simulink model "MonoRail_APU_Complete_R2016"  (R2016a)
settings: Solver=ode1  StartTime=0.0  StopTime=4.00  FixedStep=1e-6  MaxStep=1e-4  RelTol=1e-3
libraries: powerlib x67, powerlib_meascontrol x19, simulink x9, simulink_extras x3
settings Model: Creator=Hirect_MKTG  LastModifiedBy=Testinglaptop2
settings SimscapeCC: SimscapeNormalizeSystem=off

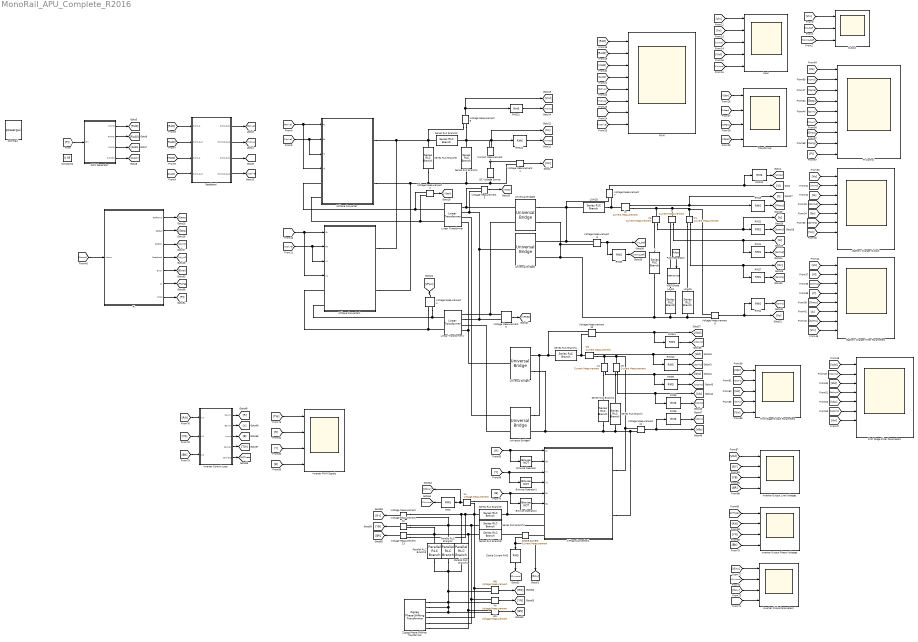
== system MonoRail_APU_Complete_R2016 ==
  3 Phase Converter : Subsystem
  3 Phase Converter1 : Subsystem
  3 Phase Converter2 : Subsystem
  BN : powerlib/Measurements/Voltage Measurement  PhasorSimulation=off  OutputType=Complex  PSBequivalent=0
  Battery Charger Filter Parameters : Scope  NumInputPorts=8
  Battery Charger Output : Scope  NumInputPorts=8
  Bitwise Operator : simulink/Logic and Bit Operations/Bitwise Operator  logicop=NOT  UseBitMask=off  BitMask=bin2dec('11011001')  BitMaskRealWorld=Stored Integer
  Bitwise Operator1 : simulink/Logic and Bit Operations/Bitwise Operator  logicop=NOT  UseBitMask=off  BitMask=bin2dec('11011001')  BitMaskRealWorld=Stored Integer
  Bitwise Operator2 : simulink/Logic and Bit Operations/Bitwise Operator  logicop=NOT  UseBitMask=off  BitMask=bin2dec('11011001')  BitMaskRealWorld=Stored Integer
  C : powerlib/Elements/Series RLC Branch  LConnTagsString=__new0  RConnTagsString=__new0  BranchType=C  Resistance=1  Inductance=1e-3  SetiL0=off  InitialCurrent=0  Capacitance=20e-3  Setx0=off  InitialVoltage=0  Measurements=None
  Choke Current RMS : powerlib_meascontrol/Measurements/RMS  TrueRMS=on  Freq=60  RMSInit=120  Ts=0
  Choke Current : powerlib/Measurements/Current Measurement  PhasorSimulation=off  OutputType=Complex  PSBequivalent=0
  Constant2 : Constant  Value=0.95  VectorParams1D=off
  Current Measurement5 : powerlib/Measurements/Current Measurement  PhasorSimulation=off  OutputType=Complex  PSBequivalent=0
  DC Voltage Source : powerlib/Electrical Sources/DC Voltage Source  Amplitude=500  Measurements=None
  Deadband : Subsystem
  First Stage Filter Parameters : Scope  NumInputPorts=8
  "First Stage Output Parameters " : Scope  NumInputPorts=5
  IGBT/Diode : powerlib/Power Electronics/IGBT//Diode  Ron=1e-3  Rs=1e5  Cs=inf  Measurements=on
  Input : Scope  NumInputPorts=5
  Inverter Choke Parameters : Scope  NumInputPorts=4
  Inverter Control Loop : Subsystem
  Inverter Output Line Voltages : Scope  NumInputPorts=4
  Inverter Output Phase Voltages : Scope  NumInputPorts=4
  Inverter PWM Signals : Scope  NumInputPorts=4
  Io : powerlib/Measurements/Current Measurement  PhasorSimulation=off  OutputType=Complex  PSBequivalent=0
  Ir{,1..5} (6 alike) : powerlib/Measurements/Current Measurement  PhasorSimulation=off  OutputType=Complex  PSBequivalent=0
  LOAD : powerlib/Elements/Series RLC Branch  LConnTagsString=__new0  RConnTagsString=__new0  BranchType=R  Resistance=58e-03  Inductance=1e-3  SetiL0=off  InitialCurrent=0  Capacitance=1e-6  Setx0=off  InitialVoltage=0  Measurements=None
  LOAD1 : powerlib/Elements/Series RLC Branch  LConnTagsString=__new0  RConnTagsString=__new0  BranchType=R  Resistance=1  Inductance=1e-3  SetiL0=off  InitialCurrent=0  Capacitance=1e-6  Setx0=off  InitialVoltage=0  Measurements=None
  LOAD3 : powerlib/Elements/Series RLC Branch  LConnTagsString=__new0  RConnTagsString=__new0  BranchType=L  Resistance=77e-03  Inductance=100e-6  SetiL0=off  InitialCurrent=0  Capacitance=1e-6  Setx0=off  InitialVoltage=0  Measurements=None
  Linear Transformer : powerlib/Elements/Linear Transformer  UNITS=SI  NominalPower=[ 50e3 50 ]  winding1=[1000 0 0]  winding2=[28.42 0 0]  ThreeWindings=on  winding3=[781 0 0]  RmLm=[inf inf]  Measurements=None  DataType=on
  Linear Transformer1 : powerlib/Elements/Linear Transformer  UNITS=SI  NominalPower=[ 50e3 50 ]  winding1=[1000 0 0]  winding2=[28.42 0 0]  ThreeWindings=on  winding3=[781 0 0]  RmLm=[inf inf]  Measurements=None  DataType=on
  Output : Scope  NumInputPorts=3
  PI : Subsystem
  PI Control : Scope  NumInputPorts=9
  PWM : Scope  NumInputPorts=8
  PWM Generator : Subsystem
  Parallel RLC Branch1 : powerlib/Elements/Parallel RLC Branch  LConnTagsString=a  RConnTagsString=__new0  BranchType=RC  Resistance=7.5  Inductance=1e-3  SetiL0=off  InitialCurrent=0  Capacitance=30e-06  Setx0=off  InitialVoltage=0  Measurements=None
  Parallel RLC Branch2 : powerlib/Elements/Parallel RLC Branch  LConnTagsString=a  RConnTagsString=__new0  BranchType=RC  Resistance=7.5  Inductance=1e-3  SetiL0=off  InitialCurrent=0  Capacitance=30e-06  Setx0=off  InitialVoltage=0  Measurements=None
  Parallel RLC Branch3 : powerlib/Elements/Parallel RLC Branch  LConnTagsString=a  RConnTagsString=__new0  BranchType=RC  Resistance=7.5  Inductance=1e-3  SetiL0=off  InitialCurrent=0  Capacitance=30e-06  Setx0=off  InitialVoltage=0  Measurements=None
  Pulse Generator : DiscretePulseGenerator  Period=1e06  PulseWidth=1e06  SampleTime=1e-06
  RMS{,1..14} (15 alike) : powerlib_meascontrol/Measurements/RMS  TrueRMS=on  Freq=60  RMSInit=120  Ts=0
  RN : powerlib/Measurements/Voltage Measurement  PhasorSimulation=off  OutputType=Complex  PSBequivalent=0
  Series RLC Branch : powerlib/Elements/Series RLC Branch  LConnTagsString=__new0  RConnTagsString=__new0  BranchType=R  Resistance=12.25  Inductance=1e-3  SetiL0=off  InitialCurrent=0  Capacitance=1e-6  Setx0=off  InitialVoltage=0  Measurements=None
  Series RLC Branch1 : powerlib/Elements/Series RLC Branch  LConnTagsString=__new0  RConnTagsString=__new0  BranchType=L  Resistance=12.25  Inductance=1e-3  SetiL0=off  InitialCurrent=0  Capacitance=1e-6  Setx0=off  InitialVoltage=0  Measurements=None
  Series RLC Branch2 : powerlib/Elements/Series RLC Branch  LConnTagsString=__new0  RConnTagsString=__new0  BranchType=C  Resistance=12.25  Inductance=1e-3  SetiL0=off  InitialCurrent=0  Capacitance=225e-6  Setx0=off  InitialVoltage=0  Measurements=None
  Series RLC Branch3 : powerlib/Elements/Series RLC Branch  LConnTagsString=__new0  RConnTagsString=__new0  BranchType=L  Resistance=12.25  Inductance=0.5e-3  SetiL0=off  InitialCurrent=0  Capacitance=1e-6  Setx0=off  InitialVoltage=0  Measurements=None
  Series RLC Branch4 : powerlib/Elements/Series RLC Branch  LConnTagsString=__new0  RConnTagsString=__new0  BranchType=RC  Resistance=0.1  Inductance=1e-3  SetiL0=off  InitialCurrent=0  Capacitance=225e-6  Setx0=off  InitialVoltage=0  Measurements=None
  Series RLC Branch5 : powerlib/Elements/Series RLC Branch  LConnTagsString=__new0  RConnTagsString=__new0  BranchType=C  Resistance=12.25  Inductance=1e-3  SetiL0=off  InitialCurrent=0  Capacitance=225e-6  Setx0=off  InitialVoltage=0  Measurements=None
  Series RLC Branch6 : powerlib/Elements/Series RLC Branch  LConnTagsString=__new0  RConnTagsString=__new0  BranchType=L  Resistance=1  Inductance=0.85e-3  SetiL0=off  InitialCurrent=0  Capacitance=1e-6  Setx0=off  InitialVoltage=0  Measurements=None
  Series RLC Branch7 : powerlib/Elements/Series RLC Branch  LConnTagsString=__new0  RConnTagsString=__new0  BranchType=L  Resistance=1  Inductance=0.85e-3  SetiL0=off  InitialCurrent=0  Capacitance=1e-6  Setx0=off  InitialVoltage=0  Measurements=None
  Series RLC Branch8 : powerlib/Elements/Series RLC Branch  LConnTagsString=__new0  RConnTagsString=__new0  BranchType=L  Resistance=1  Inductance=0.85e-3  SetiL0=off  InitialCurrent=0  Capacitance=1e-6  Setx0=off  InitialVoltage=0  Measurements=None
  Transformer : Scope  NumInputPorts=4
  Universal Bridge1 : powerlib/Power Electronics/Universal Bridge  Arms=1  SnubberResistance=1e5  SnubberCapacitance=inf  Device=Diodes  Ron=1e-3  Lon=0  ForwardVoltages="[  0  0  ]"  ForwardVoltage=0  GTOparameters=[ 10e-6 , 20e-6 ]  IGBTparameters=[ 1e-6 , 2e-6 ]  Measurements=None  Measurements_2=None  converterType=Rectifier
  Universal Bridge2 : powerlib/Power Electronics/Universal Bridge  Arms=1  SnubberResistance=1e5  SnubberCapacitance=inf  Device=Diodes  Ron=1e-3  Lon=0  ForwardVoltages="[  0  0  ]"  ForwardVoltage=0  GTOparameters=[ 10e-6 , 20e-6 ]  IGBTparameters=[ 1e-6 , 2e-6 ]  Measurements=None  Measurements_2=None  converterType=Rectifier
  Universal Bridge3 : powerlib/Power Electronics/Universal Bridge  Arms=2  SnubberResistance=1e5  SnubberCapacitance=inf  Device=Diodes  Ron=1e-3  Lon=0  ForwardVoltages="[  0  0  ]"  ForwardVoltage=0  GTOparameters=[ 10e-6 , 20e-6 ]  IGBTparameters=[ 1e-6 , 2e-6 ]  Measurements=None  Measurements_2=None  converterType=Rectifier
  Universal Bridge4 : powerlib/Power Electronics/Universal Bridge  Arms=2  SnubberResistance=1e5  SnubberCapacitance=inf  Device=Diodes  Ron=1e-3  Lon=0  ForwardVoltages="[  0  0  ]"  ForwardVoltage=0  GTOparameters=[ 10e-6 , 20e-6 ]  IGBTparameters=[ 1e-6 , 2e-6 ]  Measurements=None  Measurements_2=None  converterType=Rectifier
  VL : powerlib/Measurements/Voltage Measurement  PhasorSimulation=off  OutputType=Complex  PSBequivalent=0
  Voltage Measurement{,1..13} (14 alike) : powerlib/Measurements/Voltage Measurement  PhasorSimulation=off  OutputType=Complex  PSBequivalent=0
  YN : powerlib/Measurements/Voltage Measurement  PhasorSimulation=off  OutputType=Complex  PSBequivalent=0
  Zigzag Phase-Shifting Transformer : powerlib/Elements/Zigzag Phase-Shifting Transformer  SecondaryConnection=Yg  SetSaturation=off  SetInitialFlux=off  Measurements=None  UNITS=pu  NominalPower=[ 100e6 60]  PrimaryVoltage=10e3  SecondaryVoltage="[ 30e3  +15]"  Winding1=[ 0.002 0.08 ]  Winding2="[ 0.002  0.08 ]"  Winding3=[ 0.002 0.08 ]  RmLm=[ 500 500 ]  Rm=500  Saturation=[ 0,0 ; 0.0024,1.2 ; 1.0,1.52 ]  InitialFluxes=[0,0,0]  BreakLoop=off  DiscreteSolver=Trapezoidal iterative  DataType=off
  powergui : powerlib/powergui  Priority=1  SimulationMode=Discrete  SampleTime=1e-6  frequency=60  Iterations=50  frequencyindice=0  Pbase=100e6  ErrMax=1e-4  UnitsV=kV  UnitsW=MW  buscounter=0  FunctionMessages=off  echomessages=off  EnableUseOfTLC=off  CurrentSourceSwitches=off  DisableSnubberDevices=off  DisableRonSwitches=off  DisableVfSwitches=off  DisplayEquations=off  AutomaticDiscreteSolvers=off  SolverType=Tustin/Backward Euler (TBE)  Interpol=off  ExternalGateDelay=off  methode=off  Ts=100  x0status=blocks  SPID=on  SwTol=0  HookPort=off  NonlinearTolerance=1e-4  nMaxIteration=100  ContinueOnMaxIteration=off  RestoreLinks=warning  ResistiveCurrentMeasurement=off  Frange=[0:2:500]  Ylog=off  Xlog=on  ShowGrid=off  save=off  variable=ZData  structure=ScopeData1  ZoomFFT=on  StartTime=1  cycles=5  DisplayStyle=1  fundamental=50  FreqAxis=off  MaxFrequency=1000  frequencyindicesteady=1  RmsSteady=1  display=off
  wires:
  Current Measurement5/1 -> [Iin], RMS11/1
  Voltage Measurement1/1 -> [Vin]
  Voltage Measurement9/1 -> [Vinl], RMS12/1
  [Vo] -> PI Control/1
  [Vorms] -> PI Control/2
  [Step] -> PI Control/4
  Voltage Measurement7/1 -> [Vl], RMS10/1
  RMS10/1 -> [Vlrms]
  [Vin] -> Output/1
  [Vo_bef] -> Output/2
  [Vorms_bef] -> Output/3
  [Rdrive] -> 3 Phase Converter/4(Yb), 3 Phase Converter/1(Rt)
  [Ydrive] -> 3 Phase Converter/3(Yt), 3 Phase Converter/2(Rb)
  [Rpdrive] -> 3 Phase Converter1/1(Rt), 3 Phase Converter1/4(Yb)
  [Ypdrive] -> 3 Phase Converter1/2(Rb), 3 Phase Converter1/3(Yt)
  [Rd0] -> Deadband/1(PWM_0)
  [Rcd0] -> Deadband/2(PWM_0_C)
  [Rpd0] -> Deadband/3(PWM_P)
  [Rpcd0] -> Deadband/4(PWM_P_C)
  Deadband/1(PWM_0_D) -> [Rdrive]
  Deadband/2(PWM_0_C_D) -> [Ydrive]
  Deadband/3(PWM_P_D) -> [Rpdrive]
  Deadband/4(PWM_P_C_D) -> [Ypdrive]
  [Vin] -> Input/1
  RMS11/1 -> [Iinrms]
  [Iin] -> Input/2
  [Iinrms] -> Input/3
  RMS12/1 -> [Vinlrms]
  [Vinlrms] -> Input/5
  [Vinl] -> Input/4
  [Ramp] -> PI Control/3
  PWM Generator/1("PWM0 ") -> [Rd0]
  PWM Generator/2(PWMC) -> [Rcd0]
  PWM Generator/3(PWMP) -> [Rpd0]
  PWM Generator/4(PWMPC) -> [Rpcd0]
  PI/1(RefRamp) -> [Ramp]
  PI/2(RefSat) -> [Step]
  PI/3(RefCon) -> [ConIN]
  [Vorms] -> PI/1(Vorms)
  PI/5(Error) -> [Error]
  PI/6(PI) -> [PIorig]
  PI/7(PIsat) -> [PI]
  PI/4(Feedback) -> [Vo_un]
  [Rd0] -> PWM/1
  [Rcd0] -> PWM/2
  [Rpd0] -> PWM/3
  [Rpcd0] -> PWM/4
  [Rdrive] -> PWM/5
  [Ydrive] -> PWM/6
  [Rpdrive] -> PWM/7
  [Ypdrive] -> PWM/8
  Voltage Measurement2/1 -> [V0pri]
  Voltage Measurement3/1 -> [V0sec]
  Voltage Measurement5/1 -> [VPsec]
  Voltage Measurement4/1 -> [VPpri]
  [V0pri] -> Transformer/1
  [V0sec] -> Transformer/2
  [VPpri] -> Transformer/3
  [VPsec] -> Transformer/4
  [PI] -> PWM Generator/1(Phi)
  RMS7/1 -> [Ibrrms]
  Ir1/1 -> [Ibr], RMS7/1
  Pulse Generator/1 -> IGBT/Diode/1
  Ir/1 -> [Io], RMS1/1
  RMS1/1 -> [Iorms]
  RMS2/1 -> [Icrms]
  Ir2/1 -> [Ic], RMS2/1
  RMS3/1 -> [Ilrms]
  Io/1 -> RMS3/1, [Il]
  RMS4/1 -> [Vorms]
  Voltage Measurement6/1 -> [Vo], RMS4/1
  [Vo] -> Battery Charger Output/1
  [Vorms] -> Battery Charger Output/2
  [Io] -> Battery Charger Output/3
  [Iorms] -> Battery Charger Output/4
  [Ibr] -> Battery Charger Output/5
  [Ibrrms] -> Battery Charger Output/6
  Voltage Measurement8/1 -> [Vo_bef], RMS5/1
  RMS5/1 -> [Vorms_bef]
  [Vin] -> Battery Charger Output/7
  [Vo] -> Battery Charger Filter Parameters/1
  [Vlrms] -> Battery Charger Filter Parameters/3
  [Vl] -> Battery Charger Filter Parameters/2
  [Il] -> Battery Charger Filter Parameters/4
  [Ilrms] -> Battery Charger Filter Parameters/5
  [Ic] -> Battery Charger Filter Parameters/6
  [Icrms] -> Battery Charger Filter Parameters/7
  [Vo_un] -> PI Control/6
  [Error] -> PI Control/7
  [PIorig] -> PI Control/8
  [PI] -> PI Control/9
  [ConIN] -> PI Control/5
  Voltage Measurement10/1 -> RMS14/1, [Vdcl]
  RMS14/1 -> [Vdclrms]
  Ir3/1 -> RMS13/1, [Idcl]
  RMS13/1 -> [Idclrms]
  Ir4/1 -> RMS9/1, [Idcc]
  RMS9/1 -> [Idccrms]
  Ir5/1 -> RMS8/1, [Idc]
  RMS8/1 -> [Idcrms]
  Voltage Measurement11/1 -> RMS6/1, [Vdc]
  RMS6/1 -> [Vdcrms]
  [Vin] -> Battery Charger Filter Parameters/8
  [Vdcl] -> First Stage Filter Parameters/1
  [Vdclrms] -> First Stage Filter Parameters/2
  [Idcl] -> First Stage Filter Parameters/3
  [Idclrms] -> First Stage Filter Parameters/4
  [Idcc] -> First Stage Filter Parameters/5
  [Idccrms] -> First Stage Filter Parameters/6
  [Vin] -> First Stage Filter Parameters/7
  [Vin] -> "First Stage Output Parameters "/5
  [Vdc] -> "First Stage Output Parameters "/1
  [Vdcrms] -> "First Stage Output Parameters "/2
  [Idc] -> "First Stage Output Parameters "/3
  [Idcrms] -> "First Stage Output Parameters "/4
  Inverter Control Loop/5(Carrier2) -> [OPTheta]
  [Vlinv] -> Inverter Choke Parameters/1
  [B] -> Inverter PWM Signals/4
  [Y] -> Bitwise Operator1/1, 3 Phase Converter2/3(Yt)
  Bitwise Operator2/1 -> 3 Phase Converter2/6(Bb)
  [BN] -> Inverter Control Loop/3(In3)
  Inverter Control Loop/3(Ypwm) -> [B]
  Choke Current/1 -> Choke Current RMS/1, [Ilinv]
  [Y] -> Inverter PWM Signals/3
  [R] -> Bitwise Operator/1, 3 Phase Converter2/1(Rt)
  [TW] -> Inverter PWM Signals/1
  BN/1 -> [BN]
  [R] -> Inverter PWM Signals/2
  Inverter Control Loop/4(Carrier) -> [TW]
  [RN] -> Inverter Control Loop/1(In1)
  Inverter Control Loop/2(Bpwm) -> [Y]
  VL/1 -> [Vlinv], RMS/1
  [Ilinvrms] -> Inverter Choke Parameters/4
  RN/1 -> [RN]
  [OPTheta] -> Inverter Output Phase Voltages/1
  Voltage Measurement12/1 -> [YB]
  Bitwise Operator/1 -> 3 Phase Converter2/2(Rb)
  YN/1 -> [YN]
  [YN] -> Inverter Control Loop/2(In2)
  [BR] -> Inverter Output Line Voltages/4
  [Ilinv] -> Inverter Choke Parameters/3
  Voltage Measurement/1 -> [RY]
  [Vlinvrms] -> Inverter Choke Parameters/2
  [YB] -> Inverter Output Line Voltages/3
  Choke Current RMS/1 -> [Ilinvrms]
  Voltage Measurement13/1 -> [BR]
  [B] -> Bitwise Operator2/1, 3 Phase Converter2/5(Bt)
  Bitwise Operator1/1 -> 3 Phase Converter2/4(Yb)
  [RN] -> Inverter Output Phase Voltages/2
  [YN] -> Inverter Output Phase Voltages/3
  Inverter Control Loop/1(Rpwm) -> [R]
  [RY] -> Inverter Output Line Voltages/2
  [BN] -> Inverter Output Phase Voltages/4
  RMS/1 -> [Vlinvrms]
  [Vdcl] -> Inverter Output Line Voltages/1
  connections:
  3 Phase Converter1/RConn1 -- Series RLC Branch3/RConn1 -- Series RLC Branch5/LConn1 -- Voltage Measurement9/LConn2 -- 3 Phase Converter/RConn1
  3 Phase Converter1/RConn2 -- 3 Phase Converter/RConn2 -- Series RLC Branch5/RConn1 -- DC Voltage Source/LConn1 -- Voltage Measurement1/LConn2 -- Series RLC Branch4/RConn1
  Linear Transformer/LConn2 -- Voltage Measurement2/LConn2 -- 3 Phase Converter/LConn2
  3 Phase Converter1/LConn1 -- Linear Transformer1/LConn2 -- Voltage Measurement4/LConn2
  3 Phase Converter1/LConn2 -- Voltage Measurement4/LConn1 -- Linear Transformer1/LConn1
  3 Phase Converter/LConn1 -- Voltage Measurement2/LConn1 -- Linear Transformer/LConn1
  Series RLC Branch4/LConn1 -- Current Measurement5/RConn1 -- Series RLC Branch3/LConn1 -- Voltage Measurement9/LConn1
  DC Voltage Source/RConn1 -- Voltage Measurement1/LConn1 -- Current Measurement5/LConn1
  Universal Bridge3/LConn1 -- Linear Transformer/RConn1 -- Voltage Measurement3/LConn1
  Universal Bridge2/LConn1 -- Linear Transformer1/RConn2 -- Voltage Measurement5/LConn2 -- Voltage Measurement3/LConn2 -- Linear Transformer/RConn2
  Universal Bridge3/LConn2 -- Voltage Measurement5/LConn1 -- Linear Transformer1/RConn1
  LOAD3/RConn1 -- Universal Bridge3/RConn1 -- Voltage Measurement8/LConn1 -- Universal Bridge2/RConn1 -- Voltage Measurement7/LConn1
  Universal Bridge3/RConn2 -- C/RConn1 -- Voltage Measurement6/LConn2 -- LOAD1/RConn1 -- LOAD/RConn1 -- Universal Bridge2/RConn2 -- Voltage Measurement8/LConn2
  LOAD3/LConn1 -- Io/LConn1 -- Voltage Measurement7/LConn2
  Ir1/LConn1 -- Voltage Measurement6/LConn1 -- Ir/LConn1 -- Ir2/LConn1 -- Io/RConn1
  Ir1/RConn1 -- LOAD1/LConn1
  IGBT/Diode/RConn1 -- LOAD/LConn1
  IGBT/Diode/LConn1 -- Ir/RConn1
  Ir2/RConn1 -- C/LConn1
  Ir3/LConn1 -- Voltage Measurement10/LConn2 -- Series RLC Branch1/LConn1
  Universal Bridge4/RConn2 -- Universal Bridge1/RConn2 -- 3 Phase Converter2/RConn2 -- Voltage Measurement11/LConn2 -- Series RLC Branch/RConn1 -- Series RLC Branch2/RConn1
  Universal Bridge4/RConn1 -- Voltage Measurement10/LConn1 -- Series RLC Branch1/RConn1 -- Universal Bridge1/RConn1
  Universal Bridge1/LConn1 -- Linear Transformer/RConn4 -- Linear Transformer1/RConn4
  Universal Bridge4/LConn2 -- Linear Transformer1/RConn3
  Universal Bridge4/LConn1 -- Linear Transformer/RConn3
  Ir3/RConn1 -- 3 Phase Converter2/RConn1 -- Voltage Measurement11/LConn1 -- Ir5/LConn1 -- Ir4/LConn1
  Ir4/RConn1 -- Series RLC Branch2/LConn1
  Ir5/RConn1 -- Series RLC Branch/LConn1
  Zigzag Phase-Shifting Transformer/LConn2 -- BN/LConn2 -- Zigzag Phase-Shifting Transformer/LConn3 -- Parallel RLC Branch3/RConn1 -- Parallel RLC Branch1/RConn1 -- Parallel RLC Branch2/RConn1 -- RN/LConn2 -- YN/LConn2 -- Zigzag Phase-Shifting Transformer/LConn1
  Zigzag Phase-Shifting Transformer/LConn5 -- YN/LConn1 -- Series RLC Branch7/LConn1 -- Voltage Measurement/LConn2 -- Voltage Measurement12/LConn1 -- Parallel RLC Branch2/LConn1
  VL/LConn1 -- 3 Phase Converter2/LConn1 -- Series RLC Branch6/RConn1
  Series RLC Branch6/LConn1 -- Zigzag Phase-Shifting Transformer/LConn4 -- RN/LConn1 -- VL/LConn2 -- Voltage Measurement13/LConn2 -- Voltage Measurement/LConn1 -- Parallel RLC Branch1/LConn1
  Series RLC Branch8/LConn1 -- BN/LConn1 -- Zigzag Phase-Shifting Transformer/LConn6 -- Parallel RLC Branch3/LConn1 -- Voltage Measurement13/LConn1 -- Voltage Measurement12/LConn2
  Choke Current/RConn1 -- Series RLC Branch8/RConn1
  3 Phase Converter2/LConn2 -- Series RLC Branch7/RConn1
  3 Phase Converter2/LConn3 -- Choke Current/LConn1

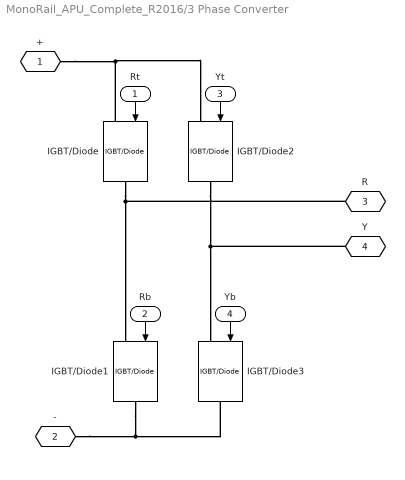
== system MonoRail_APU_Complete_R2016/3 Phase Converter ==
  Rt : Inport
  Rb : Inport  Port=2
  Yt : Inport  Port=3
  Yb : Inport  Port=4
  IGBT/Diode{,1..3} (4 alike) : powerlib/Power Electronics/IGBT//Diode  Ron=1e-3  Rs=1e5  Cs=inf  Measurements=off
  + : PMIOPort  Side=Right
  - : PMIOPort  Port=2  Side=Right
  R : PMIOPort  Port=3  Side=Left
  Y : PMIOPort  Port=4  Side=Left
  wires:
  Rt/1 -> IGBT/Diode/1
  Yb/1 -> IGBT/Diode3/1
  Rb/1 -> IGBT/Diode1/1
  Yt/1 -> IGBT/Diode2/1
  connections:
  IGBT/Diode2/RConn1 -- Y/RConn1 -- IGBT/Diode3/LConn1
  IGBT/Diode/RConn1 -- IGBT/Diode1/LConn1 -- R/RConn1
  IGBT/Diode/LConn1 -- IGBT/Diode2/LConn1 -- +/RConn1
  IGBT/Diode1/RConn1 -- -/RConn1 -- IGBT/Diode3/RConn1

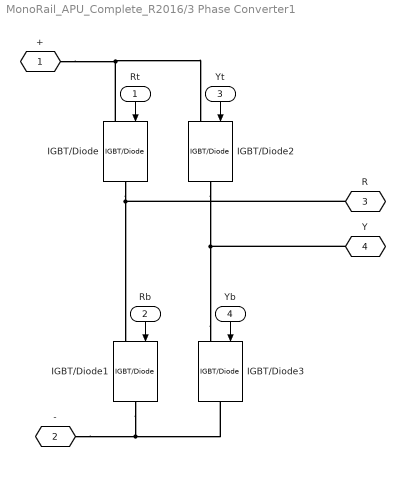
== system MonoRail_APU_Complete_R2016/3 Phase Converter1 ==
  Rt : Inport
  Rb : Inport  Port=2
  Yt : Inport  Port=3
  Yb : Inport  Port=4
  IGBT/Diode{,1..3} (4 alike) : powerlib/Power Electronics/IGBT//Diode  Ron=1e-3  Rs=1e5  Cs=inf  Measurements=off
  + : PMIOPort  Side=Right
  - : PMIOPort  Port=2  Side=Right
  R : PMIOPort  Port=3  Side=Left
  Y : PMIOPort  Port=4  Side=Left
  wires:
  Yt/1 -> IGBT/Diode2/1
  Rb/1 -> IGBT/Diode1/1
  Yb/1 -> IGBT/Diode3/1
  Rt/1 -> IGBT/Diode/1
  connections:
  IGBT/Diode3/RConn1 -- -/RConn1 -- IGBT/Diode1/RConn1
  +/RConn1 -- IGBT/Diode2/LConn1 -- IGBT/Diode/LConn1
  R/RConn1 -- IGBT/Diode1/LConn1 -- IGBT/Diode/RConn1
  IGBT/Diode3/LConn1 -- Y/RConn1 -- IGBT/Diode2/RConn1

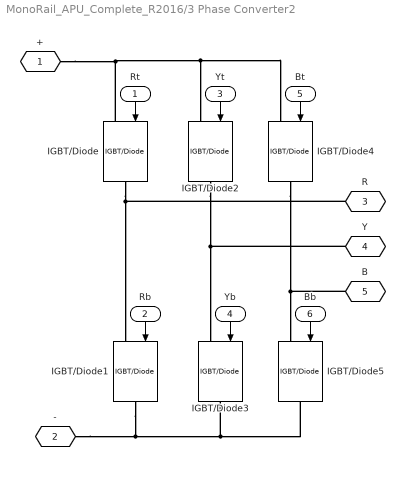
== system MonoRail_APU_Complete_R2016/3 Phase Converter2 ==
  Rt : Inport
  Rb : Inport  Port=2
  Yt : Inport  Port=3
  Yb : Inport  Port=4
  Bt : Inport  Port=5
  Bb : Inport  Port=6
  IGBT/Diode{,1..5} (6 alike) : powerlib/Power Electronics/IGBT//Diode  Ron=1e-3  Rs=1e5  Cs=inf  Measurements=off
  + : PMIOPort  Side=Right
  - : PMIOPort  Port=2  Side=Right
  R : PMIOPort  Port=3  Side=Left
  Y : PMIOPort  Port=4  Side=Left
  B : PMIOPort  Port=5  Side=Left
  wires:
  Rt/1 -> IGBT/Diode/1
  Bt/1 -> IGBT/Diode4/1
  Bb/1 -> IGBT/Diode5/1
  Yb/1 -> IGBT/Diode3/1
  Rb/1 -> IGBT/Diode1/1
  Yt/1 -> IGBT/Diode2/1
  connections:
  IGBT/Diode4/RConn1 -- B/RConn1 -- IGBT/Diode5/LConn1
  IGBT/Diode2/RConn1 -- Y/RConn1 -- IGBT/Diode3/LConn1
  IGBT/Diode/RConn1 -- IGBT/Diode1/LConn1 -- R/RConn1
  IGBT/Diode/LConn1 -- +/RConn1 -- IGBT/Diode4/LConn1 -- IGBT/Diode2/LConn1
  IGBT/Diode1/RConn1 -- -/RConn1 -- IGBT/Diode3/RConn1 -- IGBT/Diode5/RConn1

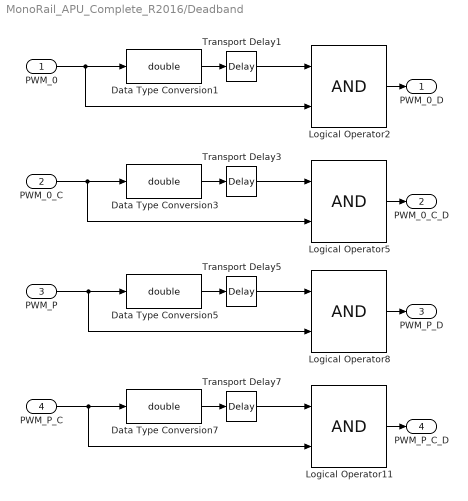
== system MonoRail_APU_Complete_R2016/Deadband ==
  PWM_0 : Inport
  PWM_0_C : Inport  Port=2
  PWM_P : Inport  Port=3
  PWM_P_C : Inport  Port=4
  Data Type Conversion{1,3,5,7} (4 alike) : DataTypeConversion  OutDataTypeStr=double
  Logical Operator{2,5,8,11} (4 alike) : Logic  AllPortsSameDT=off  OutDataTypeStr=boolean
  Transport Delay{1,3,5,7} (4 alike) : TransportDelay  DelayTime=2e-06
  PWM_0_D : Outport
  PWM_0_C_D : Outport  Port=2
  PWM_P_D : Outport  Port=3
  PWM_P_C_D : Outport  Port=4
  wires:
  Data Type Conversion1/1 -> Transport Delay1/1
  Data Type Conversion7/1 -> Transport Delay7/1
  Transport Delay3/1 -> Logical Operator5/1
  Data Type Conversion3/1 -> Transport Delay3/1
  Data Type Conversion5/1 -> Transport Delay5/1
  Transport Delay5/1 -> Logical Operator8/1
  Transport Delay1/1 -> Logical Operator2/1
  Transport Delay7/1 -> Logical Operator11/1
  PWM_P_C/1 -> Logical Operator11/2, Data Type Conversion7/1
  PWM_0/1 -> Logical Operator2/2, Data Type Conversion1/1
  Logical Operator11/1 -> PWM_P_C_D/1
  Logical Operator2/1 -> PWM_0_D/1
  PWM_0_C/1 -> Logical Operator5/2, Data Type Conversion3/1
  Logical Operator5/1 -> PWM_0_C_D/1
  Logical Operator8/1 -> PWM_P_D/1
  PWM_P/1 -> Logical Operator8/2, Data Type Conversion5/1

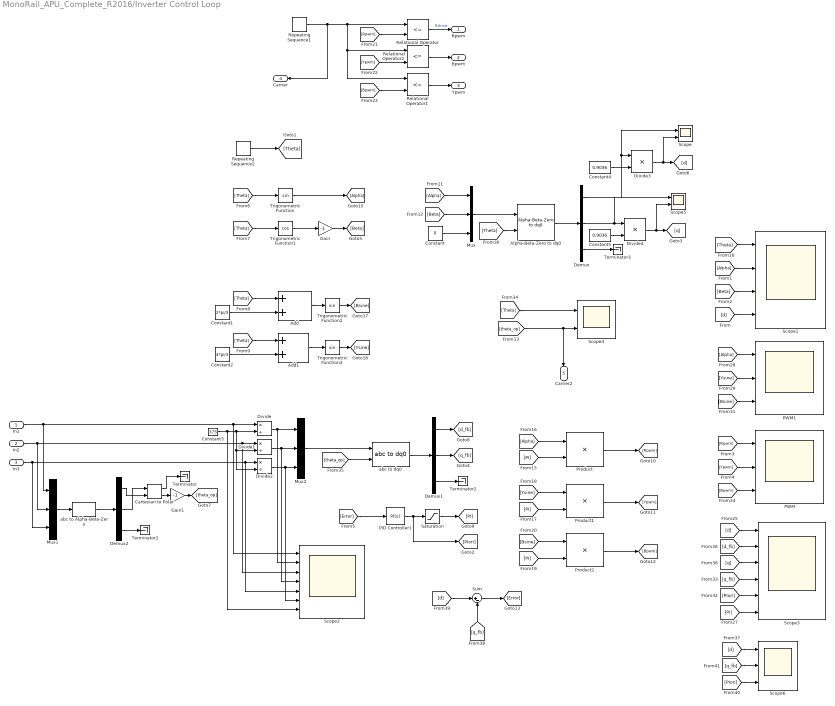
== system MonoRail_APU_Complete_R2016/Inverter Control Loop ==
  In1 : Inport
  In2 : Inport  Port=2
  In3 : Inport  Port=3
  Add : Sum
  Add1 : Sum
  Alpha-Beta-Zero to dq0 : powerlib_meascontrol/Transformations/Alpha-Beta-Zero to dq0  Alignment=90 degrees behind phase A axis
  Cartesian to Polar : simulink_extras/Transformations/Cartesian to Polar
  Constant : Constant  Value=0
  Constant1 : Constant  Value=2*pi/3
  Constant2 : Constant  Value=4*pi/3
  Constant3 : Constant  Value=375
  Constant4 : Constant  Value=0.9036
  Constant5 : Constant  Value=0.9036
  Demux : Demux  Outputs=3
  Demux1 : Demux  Outputs=3
  Demux2 : Demux  Outputs=3
  Divide : Product  Inputs=*/
  Divide1 : Product  Inputs=*/
  Divide2 : Product  Inputs=*/
  Divide3 : Product  Inputs=**
  Divide4 : Product  Inputs=**
  Gain : Gain  Gain=-1
  Gain1 : Gain  Gain=-1
  Mux : Mux  Inputs=3
  Mux1 : Mux  Inputs=3
  Mux2 : Mux  Inputs=3
  PID Controller1 : simulink/Continuous/PID Controller  Controller=PI  Form=Parallel  TimeDomain=Continuous-time  SampleTime=-1  IntegratorMethod=Forward Euler  FilterMethod=Forward Euler  ControllerParametersSource=internal  P=0.5  I=pi  D=0  UseFilter=on  N=100  InitialConditionSource=internal  InitialConditionForIntegrator=0  InitialConditionForFilter=0  DifferentiatorICPrevScaledInput=0  ExternalReset=none  TrackingMode=off  Kt=1  LimitOutput=off  UpperSaturationLimit=inf  LowerSaturationLimit=-inf  LinearizeAsGain=on  AntiWindupMode=none  Kb=1  POutMin=[]  POutMax=[]  IOutMin=[]  IOutMax=[]  DOutMin=[]  DOutMax=[]  NOutMin=[]  NOutMax=[]  SumOutMin=[]  SumOutMax=[]  SaturationOutMin=[]  SaturationOutMax=[]  PParamMin=[]  PParamMax=[]  IParamMin=[]  IParamMax=[]  DParamMin=[]  DParamMax=[]  NParamMin=[]  NParamMax=[]  KbParamMin=[]  KbParamMax=[]  KtParamMin=[]  KtParamMax=[]  KbOutMin=[]  KbOutMax=[]  KtOutMin=[]  KtOutMax=[]  IntegratorOutMin=[]  IntegratorOutMax=[]  FilterOutMin=[]  FilterOutMax=[]  SumI1OutMin=[]  SumI1OutMax=[]  SumI2OutMin=[]  SumI2OutMax=[]  SumI3OutMin=[]  SumI3OutMax=[]  SumDOutMin=[]  SumDOutMax=[]  DifferentiatorOutMin=[]  DifferentiatorOutMax=[]  IntegratorContinuousStateAttributes=''  IntegratorStateMustResolveToSignalObject=off  IntegratorRTWStateStorageClass=Auto  FilterContinuousStateAttributes=''  FilterStateMustResolveToSignalObject=off  FilterRTWStateStorageClass=Auto
  PWM : Scope  NumInputPorts=3
  PWM1 : Scope  NumInputPorts=3
  Product : Product
  Product1 : Product
  Product2 : Product
  Relational Operator : RelationalOperator  Operator=<=  OutDataTypeStr=boolean
  Relational Operator1 : RelationalOperator  Operator=<=  OutDataTypeStr=boolean
  Relational Operator2 : RelationalOperator  Operator=<=  OutDataTypeStr=boolean
  Repeating Sequence1 : simulink/Sources/Repeating Sequence  rep_seq_t=[0 1/6e03 1/3e03]  rep_seq_y=[-1 1 -1]
  Repeating Sequence2 : simulink/Sources/Repeating Sequence  rep_seq_t=[0 0.02]  rep_seq_y=[0 2*pi]
  Saturation : Saturate  UpperLimit=1  LowerLimit=-1
  Scope : Scope  NumInputPorts=2
  Scope1 : Scope  NumInputPorts=4
  Scope2 : Scope  NumInputPorts=7
  Scope3 : Scope  NumInputPorts=6
  Scope4 : Scope  NumInputPorts=2
  Scope5 : Scope  NumInputPorts=2
  Scope6 : Scope  NumInputPorts=3
  Sum : Sum  Inputs=|+-
  Terminator{,1..3} (4 alike) : Terminator
  Trigonometric Function : Trigonometry
  Trigonometric Function1 : Trigonometry  Operator=cos
  Trigonometric Function2 : Trigonometry
  Trigonometric Function3 : Trigonometry
  abc to Alpha-Beta-Zero : powerlib_meascontrol/Transformations/abc to Alpha-Beta-Zero
  abc to dq0 : powerlib_meascontrol/Transformations/abc to dq0  Alignment=Aligned with phase A axis
  Rpwm : Outport
  Bpwm : Outport  Port=2
  Ypwm : Outport  Port=3
  Carrier : Outport  Port=4
  Carrier2 : Outport  Port=5
  wires:
  Divide2/1 -> Scope2/6, Mux2/3
  In3/1 -> Mux1/3, Scope2/5, Divide2/1
  In2/1 -> Mux1/2, Scope2/3, Divide1/1
  Relational Operator/1 -> Rpwm/1  "Rdrive"
  Relational Operator2/1 -> Bpwm/1
  Relational Operator1/1 -> Ypwm/1
  [Alpha] -> Mux/1
  [Theta] -> Add/1
  Product1/1 -> [Ypwm]
  [Ysine] -> Product1/1
  [PI] -> Product1/2
  [Alpha] -> Product/1
  Mux2/1 -> abc to dq0/1
  [PI] -> Product/2
  [Ypwm] -> Relational Operator2/2
  [Rpwm] -> Relational Operator/2
  [Bsine] -> Product2/1
  [PI] -> Product2/2
  In1/1 -> Mux1/1, Scope2/1, Divide/1
  Product2/1 -> [Bpwm]
  [Bpwm] -> Relational Operator1/2
  [Beta] -> Mux/2
  Gain/1 -> [Beta]
  Trigonometric Function/1 -> [Alpha]
  Constant1/1 -> Add/2
  [Theta] -> Add1/1
  Add1/1 -> Trigonometric Function3/1
  Trigonometric Function1/1 -> Gain/1
  [Theta] -> Trigonometric Function1/1
  Constant/1 -> Mux/3
  [Theta] -> Trigonometric Function/1
  Repeating Sequence1/1 -> Carrier/1, Relational Operator1/1, Relational Operator2/1, Relational Operator/1
  Add/1 -> Trigonometric Function2/1
  [theta_op] -> abc to dq0/2
  Divide1/1 -> Scope2/4, Mux2/2
  Divide/1 -> Scope2/2, Mux2/1
  Product/1 -> [Rpwm]
  Demux1/1 -> [d_fb]
  [Theta] -> Alpha-Beta-Zero to dq0/2
  abc to dq0/1 -> Demux1/1
  Mux/1 -> Alpha-Beta-Zero to dq0/1
  Constant2/1 -> Add1/2
  [Theta] -> Scope1/1
  [Alpha] -> Scope1/2
  [Beta] -> Scope1/3
  [d] -> Scope1/4
  [Rpwm] -> PWM/1
  [Ypwm] -> PWM/2
  [Bpwm] -> PWM/3
  [d] -> Scope3/1
  [d_fb] -> Scope3/2
  [Ysine] -> PWM1/2
  [Bsine] -> PWM1/3
  [Alpha] -> PWM1/1
  Constant3/1 -> Divide2/2, Divide1/2, Divide/2, Scope2/7
  Repeating Sequence2/1 -> [Theta]
  Constant4/1 -> Divide3/2
  Divide3/1 -> Scope/2, [d]
  Demux/1 -> Scope/1, Divide3/1
  Alpha-Beta-Zero to dq0/1 -> Demux/1
  Saturation/1 -> [PI]
  [theta_op] -> Carrier2/1, Scope4/2
  [Theta] -> Scope4/1
  Trigonometric Function2/1 -> [Bsine]
  Trigonometric Function3/1 -> [Ysine]
  Mux1/1 -> abc to Alpha-Beta-Zero/1
  abc to Alpha-Beta-Zero/1 -> Demux2/1
  Demux2/2 -> Cartesian to Polar/1
  Demux2/1 -> Cartesian to Polar/2
  Demux/2 -> Scope5/1, Divide4/1
  Divide4/1 -> Scope5/2, [q]
  Constant5/1 -> Divide4/2
  Demux1/2 -> [q_fb]
  [PIori] -> Scope3/5
  [PI] -> Scope3/6
  [q_fb] -> Scope3/4
  [q] -> Scope3/3
  [PIori] -> Scope6/3
  [q_fb] -> Scope6/2
  [d] -> Scope6/1
  Cartesian to Polar/2 -> Gain1/1
  Gain1/1 -> [theta_op]
  [q_fb] -> Sum/2
  [d] -> Sum/1
  Sum/1 -> [Error]
  PID Controller1/1 -> [PIori], Saturation/1
  [Error] -> PID Controller1/1
  Cartesian to Polar/1 -> Terminator/1
  Demux2/3 -> Terminator1/1
  Demux1/3 -> Terminator2/1
  Demux/3 -> Terminator3/1

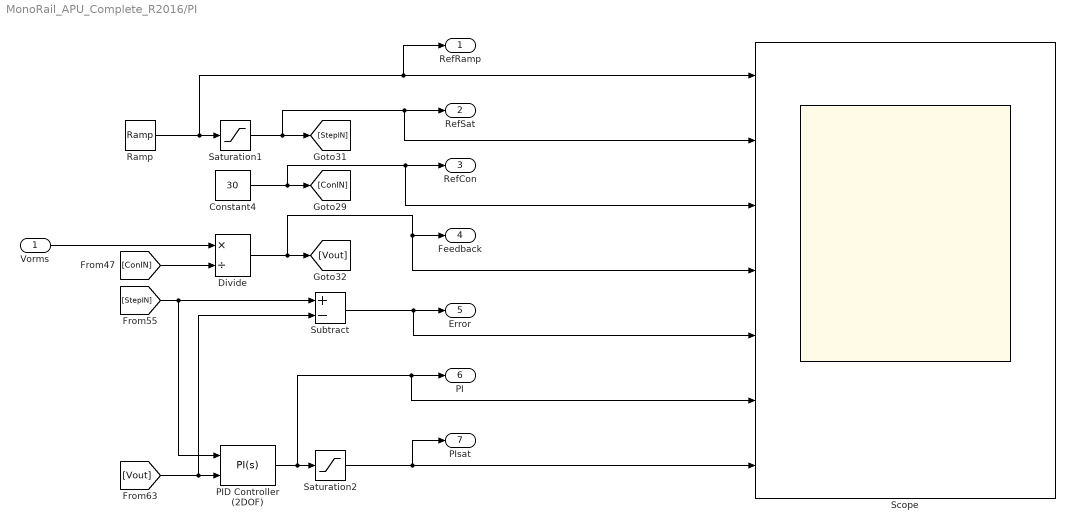
== system MonoRail_APU_Complete_R2016/PI ==
  Vorms : Inport
  Constant4 : Constant  Value=30
  Divide : Product  Inputs=*/
  PID Controller (2DOF) : simulink/Continuous/PID Controller (2DOF)  Controller=PI  Form=Parallel  TimeDomain=Continuous-time  SampleTime=-1  IntegratorMethod=Forward Euler  FilterMethod=Forward Euler  ControllerParametersSource=internal  P=0.5  I=1*pi  D=0  UseFilter=on  N=100  b=1  c=1  InitialConditionSource=internal  InitialConditionForIntegrator=0  InitialConditionForFilter=0  DifferentiatorICPrevScaledInput=0  ExternalReset=none  TrackingMode=off  Kt=1  LimitOutput=off  UpperSaturationLimit=inf  LowerSaturationLimit=-inf  LinearizeAsGain=on  AntiWindupMode=none  Kb=1  POutMin=[]  POutMax=[]  IOutMin=[]  IOutMax=[]  DOutMin=[]  DOutMax=[]  NOutMin=[]  NOutMax=[]  bOutMin=[]  bOutMax=[]  cOutMin=[]  cOutMax=[]  SumOutMin=[]  SumOutMax=[]  SaturationOutMin=[]  SaturationOutMax=[]  PParamMin=[]  PParamMax=[]  IParamMin=[]  IParamMax=[]  DParamMin=[]  DParamMax=[]  NParamMin=[]  NParamMax=[]  bParamMin=[]  bParamMax=[]  cParamMin=[]  cParamMax=[]  KbParamMin=[]  KbParamMax=[]  KtParamMin=[]  KtParamMax=[]  KbOutMin=[]  KbOutMax=[]  KtOutMin=[]  KtOutMax=[]  IntegratorOutMin=[]  IntegratorOutMax=[]  FilterOutMin=[]  FilterOutMax=[]  SumI1OutMin=[]  SumI1OutMax=[]  SumI2OutMin=[]  SumI2OutMax=[]  SumI3OutMin=[]  SumI3OutMax=[]  SumDOutMin=[]  SumDOutMax=[]  Sum1OutMin=[]  Sum1OutMax=[]  Sum2OutMin=[]  Sum2OutMax=[]  Sum3OutMin=[]  Sum3OutMax=[]  DifferentiatorOutMin=[]  DifferentiatorOutMax=[]  IntegratorContinuousStateAttributes=''  IntegratorStateMustResolveToSignalObject=off  IntegratorRTWStateStorageClass=Auto  FilterContinuousStateAttributes=''  FilterStateMustResolveToSignalObject=off  FilterRTWStateStorageClass=Auto
  Ramp : simulink/Sources/Ramp  slope=3  start=0  X0=0
  Saturation1 : Saturate  UpperLimit=0.95  LowerLimit=0.55  ZeroCross=off
  Saturation2 : Saturate  UpperLimit=inf  LowerLimit=0.05  ZeroCross=off
  Scope : Scope  NumInputPorts=7
  Subtract : Sum  Inputs=+-
  RefRamp : Outport
  RefSat : Outport  Port=2
  RefCon : Outport  Port=3
  Feedback : Outport  Port=4
  Error : Outport  Port=5
  PI : Outport  Port=6
  PIsat : Outport  Port=7
  wires:
  Constant4/1 -> RefCon/1, Scope/3, [ConIN]
  [StepIN] -> Subtract/1, PID Controller (2DOF)/1
  Ramp/1 -> RefRamp/1, Scope/1, Saturation1/1
  [ConIN] -> Divide/2
  [Vout] -> Subtract/2, PID Controller (2DOF)/2
  Vorms/1 -> Divide/1
  Subtract/1 -> Scope/5, Error/1
  Saturation2/1 -> PIsat/1, Scope/7
  Saturation1/1 -> RefSat/1, Scope/2, [StepIN]
  Divide/1 -> Scope/4, Feedback/1, [Vout]
  PID Controller (2DOF)/1 -> PI/1, Scope/6, Saturation2/1

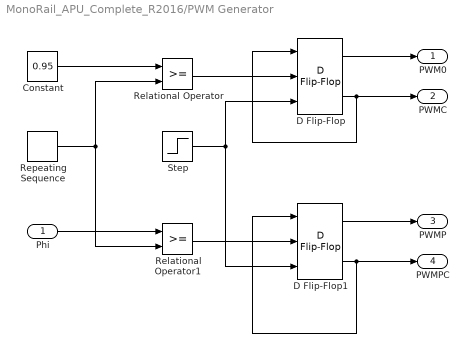
== system MonoRail_APU_Complete_R2016/PWM Generator ==
  Phi : Inport
  Constant : Constant  Value=0.95
  D Flip-Flop : simulink_extras/Flip Flops/D Flip-Flop
  D Flip-Flop1 : simulink_extras/Flip Flops/D Flip-Flop
  Relational Operator : RelationalOperator  OutDataTypeStr=boolean
  Relational Operator1 : RelationalOperator  OutDataTypeStr=boolean
  Repeating Sequence : simulink/Sources/Repeating Sequence  rep_seq_t=[0 50e-6]  rep_seq_y=[1 0]
  Step : Step  Time=1e-03  SampleTime=0
  "PWM0 " : Outport
  PWMC : Outport  Port=2
  PWMP : Outport  Port=3
  PWMPC : Outport  Port=4
  wires:
  Relational Operator1/1 -> D Flip-Flop1/2
  Repeating Sequence/1 -> Relational Operator1/2, Relational Operator/2
  Constant/1 -> Relational Operator/1
  Step/1 -> D Flip-Flop1/3, D Flip-Flop/3
  Relational Operator/1 -> D Flip-Flop/2
  D Flip-Flop1/2 -> PWMPC/1, D Flip-Flop1/1
  D Flip-Flop/2 -> PWMC/1, D Flip-Flop/1
  D Flip-Flop/1 -> "PWM0 "/1
  Phi/1 -> Relational Operator1/1
  D Flip-Flop1/1 -> PWMP/1
